simulink model "Loan_Approval"  (R2024b)
settings: Solver=VariableStepAuto  StartTime=0.0  StopTime=10.0  RelTol=1e-3
libraries: fuzblock x1

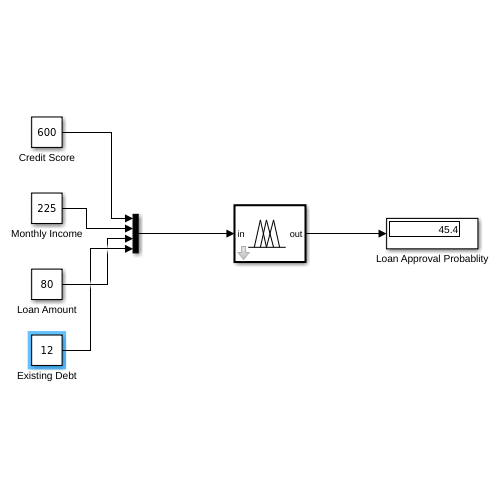
[thumbnail: Simulink's stored preview of the top-level diagram]
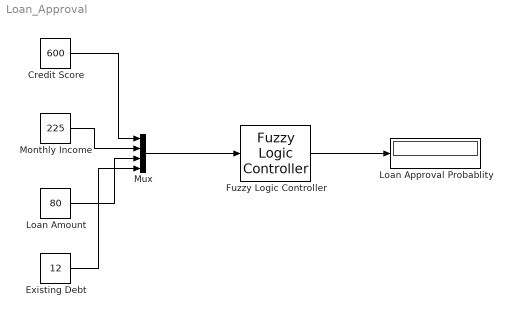
== system Loan_Approval ==
  Credit Score : Constant  Value=600
  Existing Debt : Constant  Value=12
  Fuzzy Logic Controller : fuzblock/Fuzzy Logic  Controller  FIS='Loan_Approval.fis'  OutputSampleNumber=101  DataType=double  FuzzifiedInputs=off  RuleFiringStrengths=off  RuleOutputs=off  AggregatedOutputs=off  SimulateUsing=Interpreted execution  OutOfRangeInputValueMessage=warning  NoRuleFiredMessage=warning  EmptyOutputFuzzySetMessage=warning
  Loan Amount : Constant  Value=80
  Loan Approval Probablity : Display
  Monthly Income : Constant  Value=225
  Mux : Mux
  wires:
  Mux/1 -> Fuzzy Logic Controller/1
  Credit Score/1 -> Mux/1
  Monthly Income/1 -> Mux/2
  Loan Amount/1 -> Mux/3
  Existing Debt/1 -> Mux/4
  Fuzzy Logic Controller/1 -> Loan Approval Probablity/1
